simulink library "VsrLibCoupling"  (R2019b)
settings: Solver=VariableStepAuto  StartTime=0.0  StopTime=10.0  RelTol=1e-3
libraries: autolibutils x1, autolibpowerinfoutils x1
settings Model: Creator=9bt  LastModifiedBy=4qz

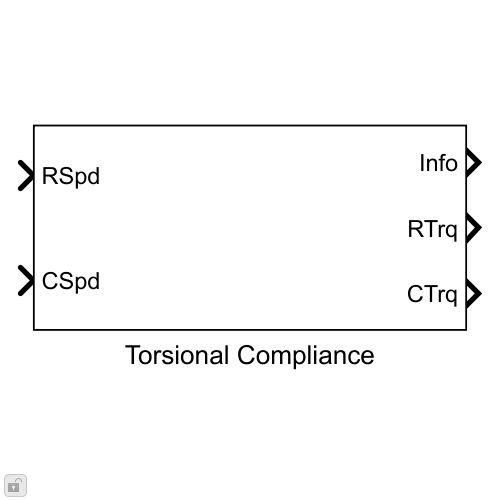
[thumbnail: Simulink's stored preview of the top-level diagram]
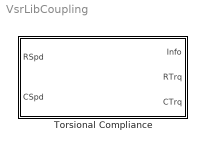
== system VsrLibCoupling ==
  Torsional Compliance : Subsystem  mask(Torsional Compliance){StiffnessCalcMethodPopup=Shaft dimensions and material properties, DampingCalcMethodPopup=Damping ratio, D_o=.05, D_i=0, L_shaft=.5, G=77e9, Jcalc=.1, zeta=.1, wn=972.0762, wd=967.2036, k=94493.2165, b=13.7472, omega_c=500, theta_0=0, omega_0=0}
      mask prompts: StiffnessCalcMethodPopup "Method for calculating stiffness:"; DampingCalcMethodPopup "Method for calculating damping:"; D_o "Outer shaft diameter, Do [m]:"; D_i "Inner shaft diameter, Di [m]:"; L_shaft "Shaft length, L_shaft [m]:"; G "Modulus of rigidity, G [Pa]:"; Jcalc "Inertia used for calculations, Jcalc [kg*m^2]:"; zeta "Damping ratio, zeta:"; wn "Calculated natural frequency, wn [rad/s]:"; wd "Calculated damped natural frequency, wd [rad/s]:"; k "Torsional stiffness, k [N*m/rad]:"; b "Torsional damping, b [N*m*s/rad]:"; omega_c "Damping cutoff frequency, omega_c [rad/s]:"; theta_0 "Initial deflection, theta_0 [rad]:"; omega_0 "Initial velocity difference, domega_0 [rad/s]:"
      mask help: Block implements a parallel spring-damper coupling.
      mask init:
      | vsr.mdl.coupling.TorsionalComplianceBlkCtrl.runInit(gcb)
      mask TypeOptions StiffnessCalcMethodPopup: None | Shaft dimensions and material properties
      mask Callback StiffnessCalcMethodPopup: vsr.mdl.coupling.TorsionalComplianceBlkCtrl.updateMask(gcb)
      mask TypeOptions DampingCalcMethodPopup: None | Damping ratio
      mask Callback DampingCalcMethodPopup: vsr.mdl.coupling.TorsionalComplianceBlkCtrl.updateMask(gcb)
      mask DialogControl ParamCalcContainer Prompt: Parameter calculation
      mask DialogControl CalcButton Prompt: Calculate Values
      mask DialogControl CalcButton Callback: vsr.mdl.coupling.TorsionalComplianceBlkCtrl.calcBlkValues(gcb)

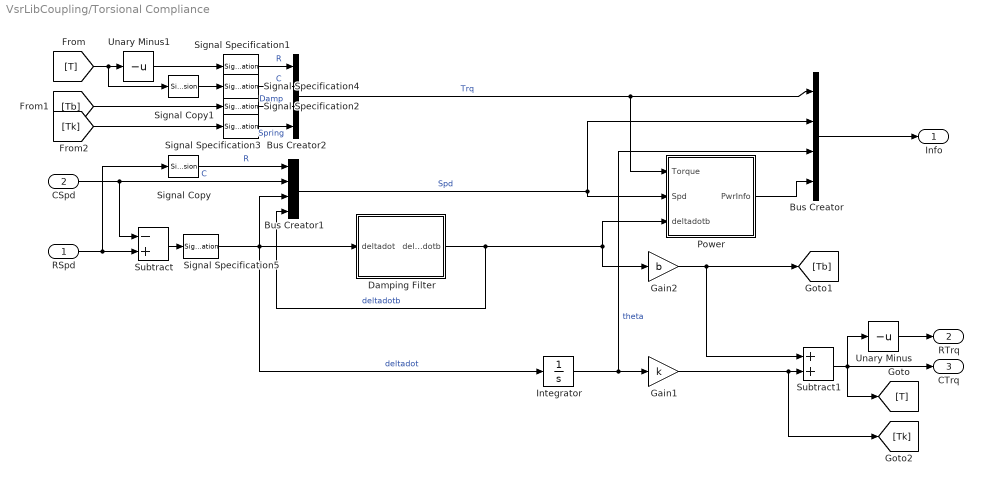
== system VsrLibCoupling/Torsional Compliance ==
  RSpd : Inport  Unit=rad/s  PortDimensions=1
  CSpd : Inport  Port=2  Unit=rad/s  PortDimensions=1
  Bus Creator : BusCreator  Inputs=4
  Bus Creator1 : BusCreator  Inputs=4
  Bus Creator2 : BusCreator  Inputs=4
  Damping Filter : Subsystem
  Gain1 : Gain  Gain=k
  Gain2 : Gain  Gain=b
  Integrator : Integrator  InitialCondition=theta_0  ZeroCross=off
  Power : Subsystem
  Signal Copy : SignalConversion  OverrideOpt=off
  Signal Copy1 : SignalConversion  OverrideOpt=off
  Signal Specification{1..4} (4 alike) : SignalSpecification  Unit=N*m
  Signal Specification5 : SignalSpecification  Unit=rad/s
  Subtract : Sum  Inputs=-+
  Subtract1 : Sum
  Unary Minus : UnaryMinus
  Unary Minus1 : UnaryMinus
  Info : Outport  VectorParamsAs1DForOutWhenUnconnected=off
  RTrq : Outport  Port=2  Unit=N*m  VectorParamsAs1DForOutWhenUnconnected=off
  CTrq : Outport  Port=3  Unit=N*m  VectorParamsAs1DForOutWhenUnconnected=off
  wires:
  Damping Filter/1(deltadotb) -> Gain2/1, Power/3(deltadotb), Bus Creator1/4  "deltadotb"
  Integrator/1 -> Gain1/1, Bus Creator/3  "theta"
  Signal Specification1/1 -> Bus Creator2/1  "R"
  Signal Copy/1 -> Bus Creator1/1  "R"
  Bus Creator2/1 -> Bus Creator/1, Power/1(Torque)  "Trq"
  Subtract1/1 -> CTrq/1, Unary Minus/1, [T]
  [T] -> Unary Minus1/1, Signal Copy1/1
  Power/1(PwrInfo) -> Bus Creator/4
  [Tb] -> Signal Specification2/1
  RSpd/1 -> Signal Copy/1, Subtract/2
  Gain1/1 -> [Tk], Subtract1/2
  Gain2/1 -> [Tb], Subtract1/1
  Unary Minus/1 -> RTrq/1
  Subtract/1 -> Signal Specification5/1
  CSpd/1 -> Bus Creator1/2, Subtract/1  "C"
  Bus Creator/1 -> Info/1
  Signal Specification4/1 -> Bus Creator2/2  "C"
  [Tk] -> Signal Specification3/1
  Signal Specification2/1 -> Bus Creator2/3  "Damp"
  Signal Specification5/1 -> Damping Filter/1(deltadot), Bus Creator1/3, Integrator/1  "deltadot"
  Signal Copy1/1 -> Signal Specification4/1
  Bus Creator1/1 -> Power/2(Spd), Bus Creator/2  "Spd"
  Unary Minus1/1 -> Signal Specification1/1
  Signal Specification3/1 -> Bus Creator2/4  "Spring"

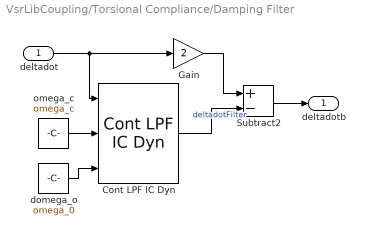
== system VsrLibCoupling/Torsional Compliance/Damping Filter ==
  deltadot : Inport
  Cont LPF IC Dyn : autolibutils/Cont LPF IC Dyn  aMode=aMode  dataType=off
  Gain : Gain  Gain=2
  Subtract2 : Sum  Inputs=+-
  domega_o : Constant  Value=omega_0
  omega_c : Constant  Value=omega_c
  deltadotb : Outport
  wires:
  Gain/1 -> Subtract2/1
  Subtract2/1 -> deltadotb/1
  deltadot/1 -> Gain/1, Cont LPF IC Dyn/1
  domega_o/1 -> Cont LPF IC Dyn/3
  Cont LPF IC Dyn/1 -> Subtract2/2  "deltadotFilter"
  omega_c/1 -> Cont LPF IC Dyn/2

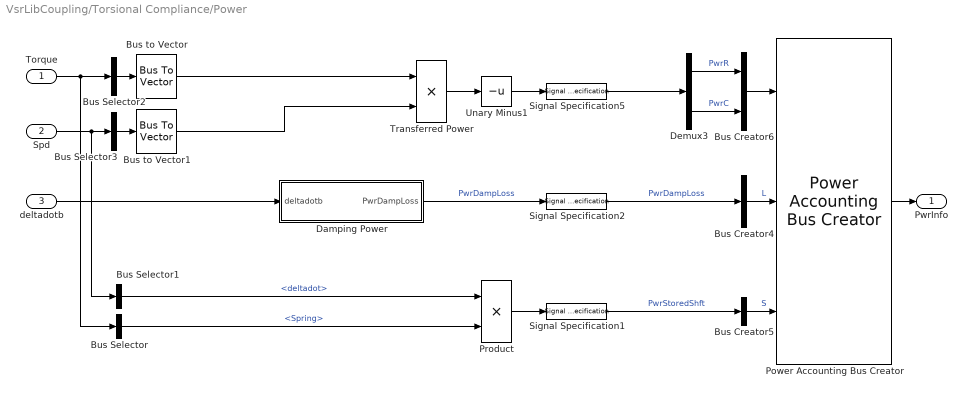
== system VsrLibCoupling/Torsional Compliance/Power ==
  Torque : Inport
  Spd : Inport  Port=2
  deltadotb : Inport  Port=3
  Bus Creator4 : BusCreator  Inputs=1
  Bus Creator5 : BusCreator  Inputs=1
  Bus Creator6 : BusCreator  Inputs=2
  Bus Selector : BusSelector  OutputSignals=Spring
  Bus Selector1 : BusSelector  OutputSignals=deltadot
  Bus Selector2 : BusSelector  OutputSignals=R,C  OutputAsBus=on
  Bus Selector3 : BusSelector  OutputSignals=R,C  OutputAsBus=on
  Bus to Vector : BusToVector
  Bus to Vector1 : BusToVector
  Damping Power : Subsystem
  Demux3 : Demux  Outputs=2
  Power Accounting Bus Creator : autolibpowerinfoutils/Power Accounting Bus Creator  AssctBlkSelPopup=Parent reference block  RefBlkName='autolibsharedcoupling/Torsional Compliance'  PwrTrnsfrdCheckBox=on  PwrNotTrnsfrdCheckBox=on  PwrStoredCheckBox=on  aMode=aMode
  Product : Product
  Signal Specification1 : SignalSpecification  Unit=W
  Signal Specification2 : SignalSpecification  Unit=W
  Signal Specification5 : SignalSpecification  Unit=W
  Transferred Power : Product
  Unary Minus1 : UnaryMinus
  PwrInfo : Outport  VectorParamsAs1DForOutWhenUnconnected=off
  wires:
  Torque/1 -> Bus Selector/1, Bus Selector2/1
  Bus Creator5/1 -> Power Accounting Bus Creator/3  "S"
  Product/1 -> Signal Specification1/1
  Bus to Vector/1 -> Transferred Power/1
  Transferred Power/1 -> Unary Minus1/1
  Power Accounting Bus Creator/1 -> PwrInfo/1
  Signal Specification2/1 -> Bus Creator4/1  "PwrDampLoss"
  Demux3/2 -> Bus Creator6/2  "PwrC"
  Bus Creator6/1 -> Power Accounting Bus Creator/1
  Demux3/1 -> Bus Creator6/1  "PwrR"
  Damping Power/1(PwrDampLoss) -> Signal Specification2/1  "PwrDampLoss"
  Bus Creator4/1 -> Power Accounting Bus Creator/2  "L"
  Bus Selector2/1 -> Bus to Vector/1
  Bus to Vector1/1 -> Transferred Power/2
  Bus Selector1/1 -> Product/1  "<deltadot>"
  Bus Selector3/1 -> Bus to Vector1/1
  Signal Specification5/1 -> Demux3/1
  Unary Minus1/1 -> Signal Specification5/1
  deltadotb/1 -> Damping Power/1(deltadotb)
  Signal Specification1/1 -> Bus Creator5/1  "PwrStoredShft"
  Spd/1 -> Bus Selector1/1, Bus Selector3/1
  Bus Selector/1 -> Product/2  "<Spring>"

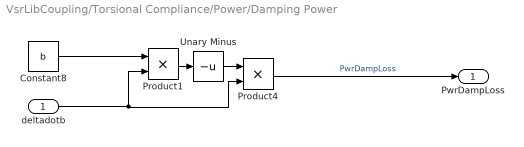
== system VsrLibCoupling/Torsional Compliance/Power/Damping Power ==
  deltadotb : Inport
  Constant8 : Constant  Value=b
  Product1 : Product
  Product4 : Product
  Unary Minus : UnaryMinus
  PwrDampLoss : Outport  VectorParamsAs1DForOutWhenUnconnected=off
  wires:
  Product1/1 -> Unary Minus/1
  Product4/1 -> PwrDampLoss/1  "PwrDampLoss"
  Unary Minus/1 -> Product4/1
  Constant8/1 -> Product1/1
  deltadotb/1 -> Product4/2, Product1/2
